simulink model "test"  (R2017b)
settings: Solver=VariableStepAuto  StartTime=0.0  StopTime=10.0  RelTol=1e-3
libraries: CarLib x1, simulink x1
settings Model: Creator=Seb  LastModifiedBy=Seb

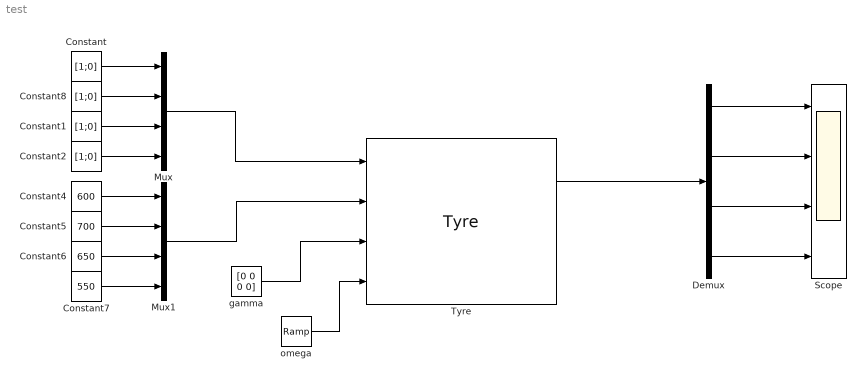
== system test ==
  Constant{,1..2,8} (4 alike) : Constant  Value=[1;0]
  Constant4 : Constant  Value=600
  Constant5 : Constant  Value=700
  Constant6 : Constant  Value=650
  Constant7 : Constant  Value=550
  Demux : Demux
  Mux : Mux
  Mux1 : Mux
  Scope : Scope  NumInputPorts=4
  "Tyre " : CarLib/Tyre  tirfilename='h.tir'
  gamma : Constant  Value=[0 0 0 0]
  omega : simulink/Sources/Ramp  slope=0.5  start=0  X0=[0 0 0 0]
  wires:
  omega/1 -> "Tyre "/4
  gamma/1 -> "Tyre "/3
  Constant1/1 -> Mux/3
  Constant/1 -> Mux/1
  Constant5/1 -> Mux1/2
  Demux/1 -> Scope/1
  Constant2/1 -> Mux/4
  Demux/4 -> Scope/4
  Constant8/1 -> Mux/2
  Mux/1 -> "Tyre "/1
  Constant6/1 -> Mux1/3
  Constant7/1 -> Mux1/4
  Demux/3 -> Scope/3
  Mux1/1 -> "Tyre "/2
  Demux/2 -> Scope/2
  Constant4/1 -> Mux1/1
  "Tyre "/1 -> Demux/1
